simulink model "designModel2"  (R2018b)
settings: Solver=ode45  StartTime=0.0  StopTime=10.0  RelTol=1e-3
values from neighbouring files (symbols this model uses):
  den1 = [tau 1]    [demo_hinf.m]
  den2 = 1    [demo_hinf.m]
  J = 0.5    [demo_hinf.m]
  num1 = 200    [demo_hinf.m]
  num2 = 0.07    [demo_hinf.m]
settings Model: ExtModeAutoUpdateStatusClock=off  Creator=biannic  LastModifiedBy=croos
settings DataIOCC: LimitDataPoints=on  SaveFormat=Array
settings OptimizationCC: BlockReduction=off  BooleanDataType=off  LifeSpan=inf
settings DebuggingCC: SaveWithParameterizedLinksMsg=none  UnderspecifiedInitializationDetection=Classic  MergeDetectMultiDrivingBlocksExec=none  SignalResolutionControl=TryResolveAllWithWarning  SFUnexpectedBacktrackingDiag=warning  SFNoUnconditionalDefaultTransitionDiag=warning  SFExecutionAtInitializationDiag=none
settings HardwareCC: ProdBitPerPointer=32  ProdBitPerSizeT=32  ProdBitPerPtrDiffT=32  ProdLargestAtomicFloat=None  ProdIntDivRoundTo=Undefined  ProdEndianess=Unspecified  ProdWordSize=32  ProdHWDeviceType=32-bit Generic  TargetUnknown=on
settings ModelReferenceCC: PropagateSignalLabelsOutOfModel=off
settings SFSimCC: SimUseLocalCustomCode=off
settings RTWCC: RTWUseLocalCustomCode=off
settings CodeAppCC: StateflowObjectComments=on
settings GRTTargetCC: TargetLangStandard=C89/C90 (ANSI)  GeneratePreprocessorConditionals=Disable all
settings ConfigComp: CovMetricSettings=dw  CovHtmlReporting=on  CovSaveCumulativeToWorkspaceVar=on  CovSaveSingleToWorkspaceVar=on  CovExternalEMLEnable=off  CovSFcnEnable=off

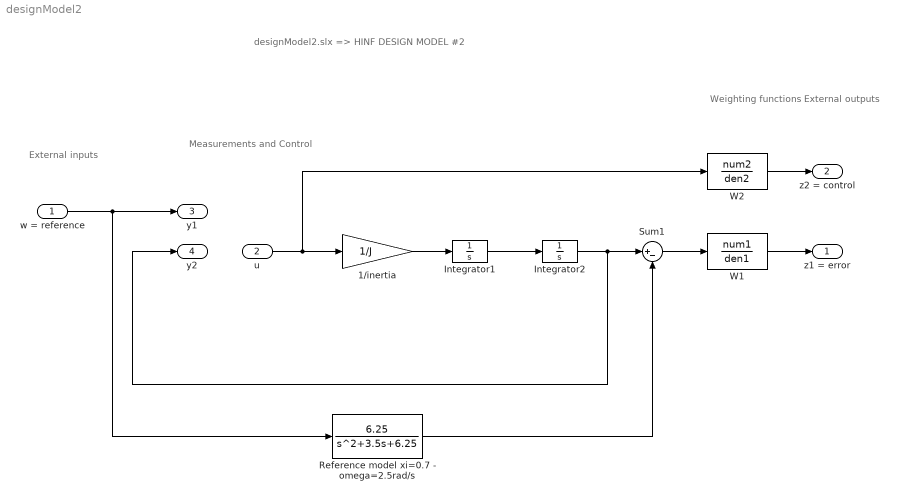
== system designModel2 ==
  note: Measurements
      | and Control
  note: External
      | outputs
  note: External
      | inputs
  note: designModel2.slx => HINF DESIGN MODEL #2
  note: Weighting
      | functions
  w = reference : Inport
  u : Inport  Port=2
  1/inertia : Gain  Gain=1/J  SaturateOnIntegerOverflow=on  OutDataTypeStr=Inherit: Same as input  ParamDataTypeStr=Inherit: Same as input
  Integrator1 : Integrator
  Integrator2 : Integrator
  Reference model xi=0.7 - omega=2.5rad/s : TransferFcn  Numerator=[6.25]  Denominator=[1 3.5 6.25]
  Sum1 : Sum  Inputs=|+-  SaturateOnIntegerOverflow=on
  W1 : TransferFcn  Numerator=num1  Denominator=den1
  W2 : TransferFcn  Numerator=num2  Denominator=den2
  z1 = error : Outport
  z2 = control : Outport  Port=2
  y1 : Outport  Port=3
  y2 : Outport  Port=4
  wires:
  Integrator1/1 -> Integrator2/1
  1/inertia/1 -> Integrator1/1
  Integrator2/1 -> y2/1, Sum1/1
  w = reference/1 -> y1/1, Reference model xi=0.7 - omega=2.5rad/s/1
  u/1 -> W2/1, 1/inertia/1
  Sum1/1 -> W1/1
  Reference model xi=0.7 - omega=2.5rad/s/1 -> Sum1/2
  W2/1 -> z2 = control/1
  W1/1 -> z1 = error/1
